simulink model "MotorDCModel_Modelado"  (R2021b)
settings: Solver=ode45  StartTime=0.0  StopTime=2.8  RelTol=1e-3  EnableMultiTasking=on
InitFcn:
  | %% Declaración de variables para sistema dinámico rotacional accionado por motor, conectado a través de banda elástica.
  | % Como referencia se pueden ver las dos fuentes a continuación:
  | % Ver: http://ctms.engin.umich.edu/CTMS/index.php?example=MotorSpeed&section=SystemModeling
  | % Ver: https://www.researchgate.net/profile/Ibraheem_Ibraheem3/post/Experiments_are_presented_assuming_nonlinear_friction_however_there_is_not_any_evidence_of_what_type_of_such_friction_is_presented_in_the_testbed/attachment/5b0e7059b53d2f63c3cef2ce/AS%3A631920186650625%401527672921693/download/Nonlinear_Modeling_and_Identification_of.pdf
  | %
  | % Estoy tomando el modelo usado en ctms, inicialmente usando sus valores.
  | % Pero añadí condiciones de fricción a partir de lo que recomienda el paper
  | % referenciado.
  | %
  | % Sin embargo, las ecuaciones del manejo de la fuerza de contacto estático,
  | % en el paper me parece qeu no toman en consideración que el signo de dicha
  | % fuerza debe ser en el sentido contrario a la aplicada y que a su vez
  | % nunca es mayor al resto de fuerzas aplicadas en reposo. Además, en
  | % simulaciones tuve problemas cuando utilicé la función signo, por
  | % excesivos cruces por cero.
  | %
  | %Por esto estoy modificando la manera en que aplico ambas fuerzas de
  | %fricción:
  | %
  | % 1: estoy manejando la fricción dinámica como T=Tdin*tanh(100*w). Esto es
  | % aprovechando tanh como una función que aproxima de forma suave la función
  | % de signo y usando 100 para hacer más rápida la transición. (Tdin es el
  | % torque de rozamiento dinámico)
  | %
  | % 2: estoy aplicando el torque de contacto como un deadzone para el torque
  | % de entrada al sistema. Y utilizando un switch dependiente, de manera que
  | % dicho deadzone solo se aplique cuando el sistema en cuestión esté en
  | % reposo.
  | 
  | L  =  0.02; % H   electric inductance
  | R  =  0.47; % Ohm  electric resistance
  | 
  | 
  | Jm  =  0.0003; % kg.m^2   moment of inertia of the rotor
  | Bm  =  0.00015; % (N.m)/(rad/s)   motor viscous friction constant
  | % Fricción dinámica y estática motor.
  | 
  | % Cambié Ke y a0M para que tengan una fórmula para lograr lo esperado en la resp a step
  | Ke =  (sqrt(1-4900*Bm*R)+1)/70;%0.1; % V/(rad/sec)  electromotive force constant
  | Kt =  Ke; % N.m/Amp  motor torque constant
  | 
  | a1M = 0;%0.1; % N.m min torque para iniciar mov en el motor.
  | a0M = 3/7*Kt/R%0.7*a1M; % (N.m)/(rad/s) torque de fricción motor debido a la velocidad
settings Model: Creator=amind  LastModifiedBy=new
settings SolverCC: AlgebraicLoopSolver=TrustRegion
settings DataIOCC: LimitDataPoints=on  SaveFormat=Array  ReturnWorkspaceOutputs=off
settings OptimizationCC: LifeSpan=inf
settings DebuggingCC: SFUnexpectedBacktrackingDiag=warning  SFNoUnconditionalDefaultTransitionDiag=warning  SFExecutionAtInitializationDiag=none  SFMachineParentedDataDiag=warning  ArithmeticOperatorsInVariantConditions=warning
settings HardwareCC: ProdBitPerPointer=32  ProdBitPerSizeT=32  ProdBitPerPtrDiffT=32  ProdLargestAtomicFloat=None  ProdIntDivRoundTo=Undefined  ProdEndianess=Unspecified  ProdWordSize=32  ProdHWDeviceType=32-bit Generic
settings ModelReferenceCC: PropagateSignalLabelsOutOfModel=off
settings SFSimCC: SimUseLocalCustomCode=off  CustomCodeUndefinedFunction=UseInterfaceOnly
settings RTWCC: RTWUseLocalCustomCode=off
settings CodeAppCC: StateflowObjectComments=on
settings GRTTargetCC: TargetLangStandard=C89/C90 (ANSI)
settings ConfigComp: CovMetricSettings=dw  CovSaveCumulativeToWorkspaceVar=on  CovSaveSingleToWorkspaceVar=on  CovExternalEMLEnable=off

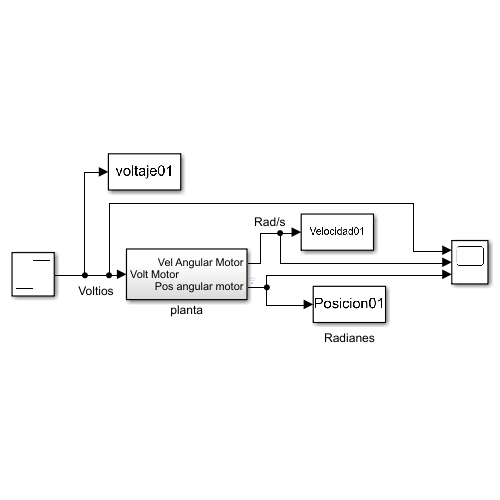
[thumbnail: Simulink's stored preview of the top-level diagram]
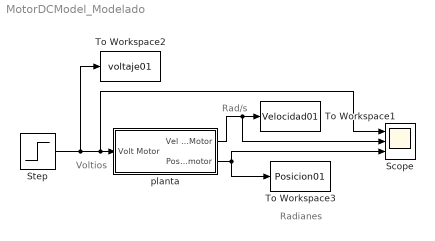
== system MotorDCModel_Modelado ==
  note: Voltios
  note: Rad/s
  note: Radianes
  Scope : Scope  NumInputPorts=3
  Step : Step  After=3  SampleTime=0
  To Workspace1 : ToWorkspace  VariableName=Velocidad01  SaveFormat=Timeseries  SampleTime=-1
  To Workspace2 : ToWorkspace  VariableName=voltaje01  SaveFormat=Timeseries  SampleTime=-1
  To Workspace3 : ToWorkspace  VariableName=Posicion01  SaveFormat=Timeseries  SampleTime=-1
  planta : Subsystem
  wires:
  planta/2(Pos angular motor) -> To Workspace3/1, Scope/3
  planta/1(Vel Angular Motor) -> To Workspace1/1, Scope/2
  Step/1 -> Scope/1, planta/1(Volt Motor), To Workspace2/1

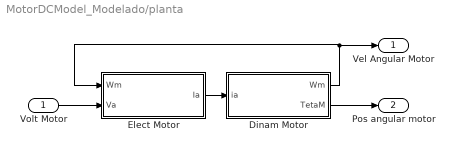
== system MotorDCModel_Modelado/planta ==
  Volt Motor : Inport
  Dinam Motor : Subsystem
  Elect Motor : Subsystem
  Vel Angular Motor : Outport
  Pos angular motor : Outport  Port=2
  wires:
  Elect Motor/1(Ia) -> Dinam Motor/1(ia)
  Dinam Motor/1(Wm) -> Vel Angular Motor/1, Elect Motor/1(Wm)
  Dinam Motor/2(TetaM) -> Pos angular motor/1
  Volt Motor/1 -> Elect Motor/2(Va)

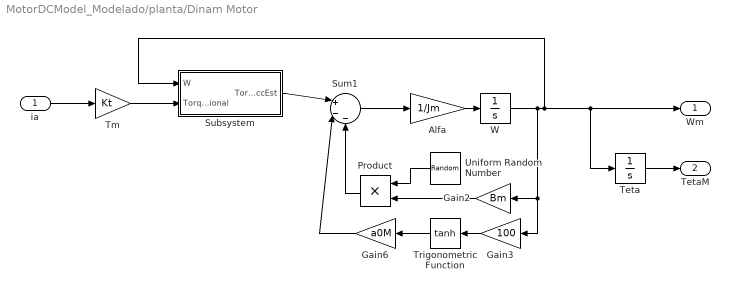
== system MotorDCModel_Modelado/planta/Dinam Motor ==
  ia : Inport
  Alfa : Gain  Gain=1/Jm
  Gain2 : Gain  Gain=Bm
  Gain3 : Gain  Gain=100
  Gain6 : Gain  Gain=a0M
  Product : Product
  Subsystem : Subsystem
  Sum1 : Sum  Inputs=|+--
  Teta : Integrator
  Tm : Gain  Gain=Kt
  Trigonometric Function : Trigonometry  Operator=tanh
  Uniform Random Number : UniformRandomNumber  Minimum=.8  Maximum=1.2  SampleTime=0.1
  W : Integrator
  Wm : Outport
  TetaM : Outport  Port=2
  wires:
  Alfa/1 -> W/1
  Sum1/1 -> Alfa/1
  W/1 -> Subsystem/1(W), Wm/1, Teta/1, Gain3/1, Gain2/1
  Gain6/1 -> Sum1/2
  ia/1 -> Tm/1
  Teta/1 -> TetaM/1
  Tm/1 -> Subsystem/2(TorqPosicional)
  Subsystem/1(TorqFriccEst) -> Sum1/1
  Gain2/1 -> Product/2
  Trigonometric Function/1 -> Gain6/1
  Gain3/1 -> Trigonometric Function/1
  Uniform Random Number/1 -> Product/1
  Product/1 -> Sum1/3

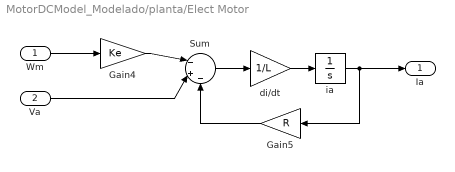
== system MotorDCModel_Modelado/planta/Elect Motor ==
  Wm : Inport
  Va : Inport  Port=2
  Gain4 : Gain  Gain=Ke
  Gain5 : Gain  Gain=R
  Sum : Sum  Inputs=|-+-
  di/dt : Gain  Gain=1/L
  ia : Integrator
  Ia : Outport
  wires:
  Sum/1 -> di/dt/1
  di/dt/1 -> ia/1
  Gain5/1 -> Sum/3
  Va/1 -> Sum/2
  Wm/1 -> Gain4/1
  Gain4/1 -> Sum/1
  ia/1 -> Ia/1, Gain5/1

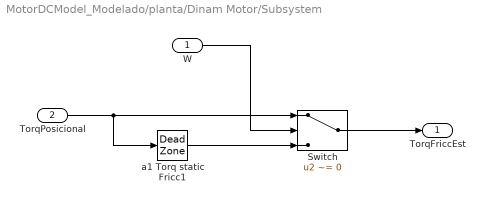
== system MotorDCModel_Modelado/planta/Dinam Motor/Subsystem ==
  W : Inport
  TorqPosicional : Inport  Port=2
  Switch : Switch  Criteria=u2 ~= 0
  a1 Torq static Fricc1 : DeadZone  LowerValue=-a1M  UpperValue=a1M  SaturateOnIntegerOverflow=on
  TorqFriccEst : Outport
  wires:
  Switch/1 -> TorqFriccEst/1
  TorqPosicional/1 -> a1 Torq static Fricc1/1, Switch/1
  W/1 -> Switch/2
  a1 Torq static Fricc1/1 -> Switch/3
